simulink model "power_supply_test"  (R2025b)
settings: Solver=FixedStepAuto  StartTime=0.0  StopTime=2  RelTol=1e-3
model workspace (MAT data in the model file):
  Ap = 0.0314
  Ct = 2.4e-12
  Fforce = 90000
  GateChoice = "linear"
  Gmass = 9000
  K1 = 221320
  K2 = 0.00072
  Kc = 1.68e-09
  Kq = 1.63
  Ksvl = 0.0276
  Ksvr = 0.04
  U_PhaseRMS = 243
  Ve = 0.11304
  Xd = 0.003
  Xmax = 0.006
  Xmin = -0.004
  beta_e = 700000000
  delay_t = 1e-06
  dl = -0.014
  dr = 0.014
  k = 0.15
  lambda = 2
  rd = 0.0004
undefined symbols (not defined in the file or in its folder): R_rms, Rn_SNR, Ts_meas
libraries: ee_lib x13, nesl_utility x4, fl_lib x3, eeRmsMeasurement x3, simulink x1
settings Model: DataDictionary=ctrlSys.sldd  Creator=LYG  LastModifiedBy=LYG
settings SolverCC: ZeroCrossControl=DisableAll

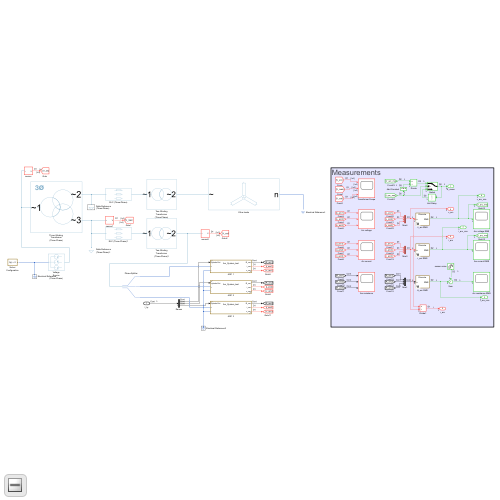
[thumbnail: Simulink's stored preview of the top-level diagram]
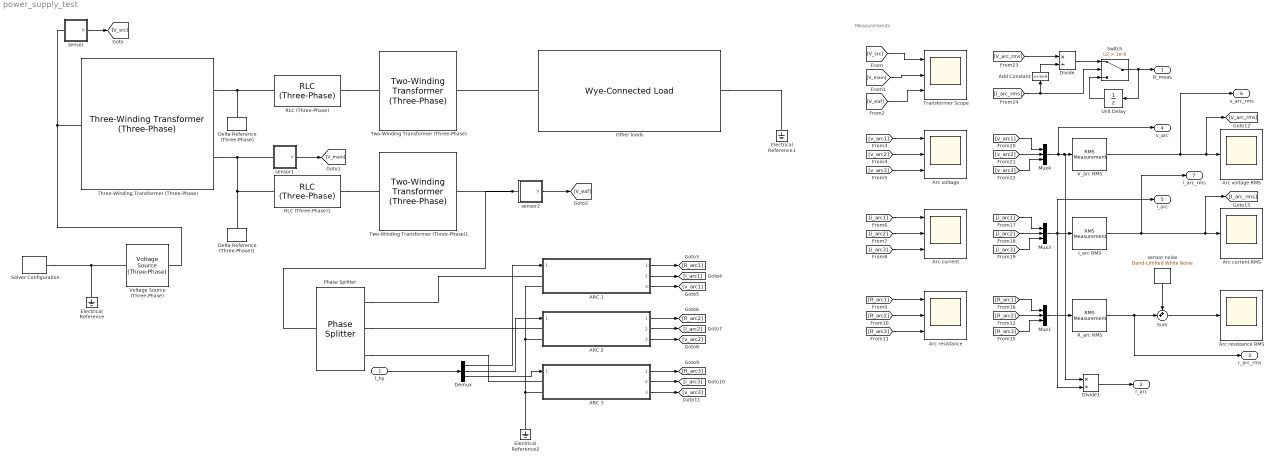
== system power_supply_test ==
  note: Measurements
  l_hy : Inport
  ARC 1 : Subsystem  ReferencedSubsystem=Arc_System_test
  ARC 2 : Subsystem  ReferencedSubsystem=Arc_System_test
  ARC 3 : Subsystem  ReferencedSubsystem=Arc_System_test
  Add Constant : Bias  Bias=1e-6  SaturateOnIntegerOverflow=off
  Arc current : Scope  NumInputPorts=3
      settings: ActiveDisplayYMinimum=-41973.164268779663  ActiveDisplayYMaximum=41974.004776580055  DataLoggingVariableName=ScopeData2
  Arc current RMS : Scope
      settings: ActiveDisplayYMinimum=-3055.4847803654839  ActiveDisplayYMaximum=27499.363023289359  DataLoggingVariableName=ScopeData7
  Arc resistance : Scope  NumInputPorts=3
      settings: ActiveDisplayYMinimum=-0.1125194623785952  ActiveDisplayYMaximum=1.0569916577736953  DataLoggingVariableName=ScopeData3
  Arc resistance RMS : Scope
      settings: ActiveDisplayYMinimum=0.04995143409404143  ActiveDisplayYMaximum=0.074820253608208473  DataLoggingVariableName=ScopeData4
  Arc voltage : Scope  NumInputPorts=3
      settings: ActiveDisplayYMinimum=351.3925306602107  ActiveDisplayYMaximum=415.43919686304929
  Arc voltage RMS : Scope
      settings: ActiveDisplayYMinimum=-47.465203373542423  ActiveDisplayYMaximum=427.18683036188185  DataLoggingVariableName=ScopeData8
  Delta Reference (Three-Phase) : ee_lib/Connectors & References/Delta Reference (Three-Phase)
      settings: InternalSimscapePortConfiguration="{\"Bottom\":[],\"Left\":[{\"id\":\"N\",\"label\":\"~\",\"type\":\"foundation.electrical.three_phase\"}],\"Right\":[],\"Top\":[]}"
  Delta Reference (Three-Phase)1 : ee_lib/Connectors & References/Delta Reference (Three-Phase)
      settings: InternalSimscapePortConfiguration="{\"Bottom\":[],\"Left\":[{\"id\":\"N\",\"label\":\"~\",\"type\":\"foundation.electrical.three_phase\"}],\"Right\":[],\"Top\":[]}"
  Demux : Demux  Outputs=3
  Divide : Product  Inputs=*/  OutMin=0
  Divide1 : Product  Inputs=*/
  Electrical Reference : fl_lib/Electrical/Electrical Elements/Electrical Reference
  Electrical Reference1 : fl_lib/Electrical/Electrical Elements/Electrical Reference
  Electrical Reference2 : fl_lib/Electrical/Electrical Elements/Electrical Reference
  I_arc RMS : eeRmsMeasurement/RMS Measurement  LabelModeActiveChoice=Total  F=f  SpecifyHarmonics=off  K=[0 1 2]  Ts=Ts_meas
      settings: LibrarySourceBlock=|
      | ee_sl_lib/Measurements/RMS
      | Measurement
  Mux1 : Mux  Inputs=3
  Mux3 : Mux  Inputs=3
  Mux4 : Mux  Inputs=3
  Other loads : ee_lib/Passive/RLC Assemblies/Wye-Connected Load  port_option=ee.enum.threePhasePort.composite  parameterization=ee.enum.rlc.parameterization.ratedpower  component_structure=ee.enum.rlc.structure.R  component_structure_PQ=ee.enum.rlc.structure.SeriesRLC  R=1 Ohm  L=1e-3 H  C=1e-6 F  VRated=6000 V  FRated=f Hz  P=10000 W  Qpos=100 A*V  Qneg=-1e2 A*V  R_parasitic=0 Ohm  G_parasitic=0 1/Ohm  R_parasitic_PQ=0 Ohm  G_parasitic_PQ=0 1/Ohm  Vmag0=24e3 V  Vang0=0 deg  Freq0=60 Hz  IL_specify=off  IL_priority=High  IL=[0, 0, 0] A  IL_nominal_specify=off  IL_nominal_value=1  IL_nominal_unit=A  VC_specify=off  VC_priority=High  VC=[0, 0, 0] V  VC_nominal_specify=off  VC_nominal_value=1  VC_nominal_unit=V
  Phase Splitter : ee_lib/Connectors & References/Phase Splitter
  RLC (Three-Phase) : ee_lib/Passive/RLC Assemblies/RLC (Three-Phase)  port_option=ee.enum.threePhasePort.composite  component_structure=ee.enum.rlc.structure.R  R=0.256 Ohm  L=8e-3 H  C=1e-6 F  R_parasitic=0 Ohm  G_parasitic=0 1/Ohm  IL_specify=off  IL_priority=High  IL=[0, 0, 0] A  IL_nominal_specify=off  IL_nominal_value=1  IL_nominal_unit=A  VC_specify=off  VC_priority=High  VC=[0, 0, 0] V  VC_nominal_specify=off  VC_nominal_value=1  VC_nominal_unit=V
      settings: InternalSimscapePortConfiguration="{\"Bottom\":[],\"Left\":[{\"id\":\"N1\",\"label\":\"~1\",\"type\":\"foundation.electrical.three_phase\"}],\"Right\":[{\"id\":\"N2\",\"label\":\"~2\",\"type\":\"foundation.electrical.three_phase\"}],\"Top\":[]}"
  RLC (Three-Phase)1 : ee_lib/Passive/RLC Assemblies/RLC (Three-Phase)  port_option=ee.enum.threePhasePort.composite  component_structure=ee.enum.rlc.structure.R  R=0.256 Ohm  L=8e-3 H  C=1e-6 F  R_parasitic=0 Ohm  G_parasitic=0 1/Ohm  IL_specify=off  IL_priority=High  IL=[0, 0, 0] A  IL_nominal_specify=off  IL_nominal_value=1  IL_nominal_unit=A  VC_specify=off  VC_priority=High  VC=[0, 0, 0] V  VC_nominal_specify=off  VC_nominal_value=1  VC_nominal_unit=V
      settings: InternalSimscapePortConfiguration="{\"Bottom\":[],\"Left\":[{\"id\":\"N1\",\"label\":\"~1\",\"type\":\"foundation.electrical.three_phase\"}],\"Right\":[{\"id\":\"N2\",\"label\":\"~2\",\"type\":\"foundation.electrical.three_phase\"}],\"Top\":[]}"
  R_arc RMS : eeRmsMeasurement/RMS Measurement  LabelModeActiveChoice=Total  F=f  SpecifyHarmonics=off  K=[0 1 2]  Ts=Ts_meas
      settings: LibrarySourceBlock=|
      | ee_sl_lib/Measurements/RMS
      | Measurement
  Solver Configuration : nesl_utility/Solver Configuration  PhysicalDomain=network_engine_domain  SubClassName=solver  LeftPortType=input  RightPortType=generic  Tones=[]  Harmonics=[]  SimulateNoise=off  Profile=off  UseLocalSampling=off  EnableSwitchedLinearOptims=on  FrequencyDomain=off  UseCCode=off  RelTol=0.001  AbsTol=0.001  MinStep=1e-09  ToWorkspace=off  RevertToSquareIcSolve=off  NumHomotopyIterations=100  PhasorMode=off  PhasorModeNumHarmonics=1  ConsistencySolver=NEWTON_XTOL_AFTER_FTOL  IndexReductionMethod=DerivativeReplacement  DoDC=off  ResidualTolerance=1e-09  ConsistencyTolSource=GLOBAL  ConsistencyAbsTol=0.001  ConsistencyRelTol=0.001  ConsistencyTolFactor=0.001  UseLocalSolver=on  LocalSolverChoice=NE_BACKWARD_EULER_ADVANCER  ResolveIndetEquations=on  FunctionEvalNumThread=1  LocalSolverSampleTime=Ts_local  DoFixedCost=off  MaxNonlinIter=5  MaxModeIter=2  ComputeImpulses=off  ImpulseIterations=2  LinearAlgebra=auto  LinearAlgebraNumThread=0  EquationFormulation=NE_TIME_EF  DelaysMemoryBudget=1024  AutomaticFiltering=on  FilteringTimeConstant=0.001  PartitionStorageMethod=AS_NEEDED  PartitionMemoryBudget=1024  PartitionMethod=ROBUST  MultibodyUseLocalSolver=off  MultibodyLocalSolverChoice=ODE1  MultibodyLocalSolverSampleTime=0.001
  Sum : Sum  Inputs=++|
  Switch : Switch  Criteria=u2 > Threshold  Threshold=1e-6  SaturateOnIntegerOverflow=off  InputSameDT=off
  Three-Winding Transformer (Three-Phase) : ee_lib/Passive/Transformers/Three-Winding Transformer (Three-Phase)  SRated=100e6 A*V  FRated=f Hz  Winding1Connection=ee.enum.windingconnection.delta1  VRated1=110e3 V  Winding2Connection=ee.enum.windingconnection.delta1  VRated2=3.5e3 V  Winding3Connection=ee.enum.windingconnection.delta1  VRated3=3.5e3 V  CoreType=ee.enum.coretype.threelimb  pu_Rw1=0.01  pu_Rw2=0.01  pu_Rw3=0.01  leakage_reactance_option=ee.enum.transformer_leakage.exclude  pu_Xl1=0.05  pu_Xl2=0.05  pu_Xl3=0.05  magnetizing_resistance_option=ee.enum.transformer_magnetizingResistance.exclude  pu_Rm=500  magnetizing_reactance_option=ee.enum.transformer_magnetizingReactance.exclude  saturation_option=ee.enum.transformer_saturation.exclude  pu_Xm=500  current_data=[0, .002, 1, 2]  magnetic_flux_data=[0, 1.2, 1.5, 1.51]  pu_X0=0.5  i1_specify=off  i1_priority=None  i1=[0, 0, 0] A  i1_nominal_specify=off  i1_nominal_value=1  i1_nominal_unit=A  i2_specify=off  i2_priority=None  i2=[0, 0, 0] A  i2_nominal_specify=off  i2_nominal_value=1  i2_nominal_unit=A  i3_specify=off  i3_priority=None  i3=[0, 0, 0] A  i3_nominal_specify=off  i3_nominal_value=1  i3_nominal_unit=A  phi_specify=off  phi_priority=None  phi=[0, 0, 0]  phi_nominal_specify=off  phi_nominal_value=1  phi_nominal_unit=1  power_dissipated_specify=off  power_dissipated_priority=None  power_dissipated=0 W  power_dissipated_nominal_specify=off  power_dissipated_nominal_value=1  power_dissipated_nominal_unit=W
      settings: InternalSimscapePortConfiguration="{\"Bottom\":[],\"Left\":[{\"id\":\"N1\",\"label\":\"~1\",\"type\":\"foundation.electrical.three_phase\"}],\"Right\":[{\"id\":\"N2\",\"label\":\"~2\",\"type\":\"foundation.electrical.three_phase\"},{\"id\":\"N3\",\"label\":\"~3\",\"type\":\"foundation.electrical.three_phase\"}],\"Top\":[]}"
  Transformer Scope : Scope  NumInputPorts=3
      settings: ActiveDisplayYMinimum=-194454.28422245517  ActiveDisplayYMaximum=194453.63939169198
  Two-Winding Transformer (Three-Phase) : ee_lib/Passive/Transformers/Two-Winding Transformer (Three-Phase)  SRated=100e6 A*V  FRated=f Hz  Winding1Connection=ee.enum.windingconnection.delta1  VRated1=735000 V  Winding2Connection=ee.enum.windingconnection.Y  VRated2=8820 V  CoreType=ee.enum.coretype.threelimb  pu_Rw1=0.01  pu_Rw2=0.01  leakage_reactance_option=ee.enum.transformer_leakage.exclude  pu_Xl1=0.05  pu_Xl2=0.05  magnetizing_resistance_option=ee.enum.transformer_magnetizingResistance.exclude  pu_Rm=500  magnetizing_reactance_option=ee.enum.transformer_magnetizingReactance.exclude  saturation_option=ee.enum.transformer_saturation.exclude  pu_Xm=500  current_data=[0, .002, 1, 2]  magnetic_flux_data=[0, 1.2, 1.5, 1.51]  pu_X0=0.5  i1_specify=off  i1_priority=None  i1=[0, 0, 0] A  i1_nominal_specify=off  i1_nominal_value=1  i1_nominal_unit=A  i2_specify=off  i2_priority=None  i2=[0, 0, 0] A  i2_nominal_specify=off  i2_nominal_value=1  i2_nominal_unit=A  phi_specify=off  phi_priority=None  phi=[0, 0, 0]  phi_nominal_specify=off  phi_nominal_value=1  phi_nominal_unit=1  power_dissipated_specify=off  power_dissipated_priority=None  power_dissipated=0 W  power_dissipated_nominal_specify=off  power_dissipated_nominal_value=1  power_dissipated_nominal_unit=W
      settings: InternalSimscapePortConfiguration="{\"Bottom\":[],\"Left\":[{\"id\":\"N1\",\"label\":\"~1\",\"type\":\"foundation.electrical.three_phase\"}],\"Right\":[{\"id\":\"N2\",\"label\":\"~2\",\"type\":\"foundation.electrical.three_phase\"}],\"Top\":[]}"
  Two-Winding Transformer (Three-Phase)1 : ee_lib/Passive/Transformers/Two-Winding Transformer (Three-Phase)  SRated=100e6 A*V  FRated=f Hz  Winding1Connection=ee.enum.windingconnection.delta1  VRated1=3.5e3 V  Winding2Connection=ee.enum.windingconnection.delta1  VRated2=580 V  CoreType=ee.enum.coretype.threelimb  pu_Rw1=0.01  pu_Rw2=0.01  leakage_reactance_option=ee.enum.transformer_leakage.exclude  pu_Xl1=0.05  pu_Xl2=0.05  magnetizing_resistance_option=ee.enum.transformer_magnetizingResistance.exclude  pu_Rm=500  magnetizing_reactance_option=ee.enum.transformer_magnetizingReactance.exclude  saturation_option=ee.enum.transformer_saturation.exclude  pu_Xm=500  current_data=[0, .002, 1, 2]  magnetic_flux_data=[0, 1.2, 1.5, 1.51]  pu_X0=0.5  i1_specify=off  i1_priority=None  i1=[0, 0, 0] A  i1_nominal_specify=off  i1_nominal_value=1  i1_nominal_unit=A  i2_specify=off  i2_priority=None  i2=[0, 0, 0] A  i2_nominal_specify=off  i2_nominal_value=1  i2_nominal_unit=A  phi_specify=off  phi_priority=None  phi=[0, 0, 0]  phi_nominal_specify=off  phi_nominal_value=1  phi_nominal_unit=1  power_dissipated_specify=off  power_dissipated_priority=None  power_dissipated=0 W  power_dissipated_nominal_specify=off  power_dissipated_nominal_value=1  power_dissipated_nominal_unit=W
      settings: InternalSimscapePortConfiguration="{\"Bottom\":[],\"Left\":[{\"id\":\"N1\",\"label\":\"~1\",\"type\":\"foundation.electrical.three_phase\"}],\"Right\":[{\"id\":\"N2\",\"label\":\"~2\",\"type\":\"foundation.electrical.three_phase\"}],\"Top\":[]}"
  Unit Delay : UnitDelay  SampleTime=-1  HasFrameUpgradeWarning=on
  V_arc RMS : eeRmsMeasurement/RMS Measurement  LabelModeActiveChoice=Total  F=f  SpecifyHarmonics=off  K=[0 1 2]  Ts=Ts_meas
      settings: LibrarySourceBlock=|
      | ee_sl_lib/Measurements/RMS
      | Measurement
  Voltage Source (Three-Phase) : ee_lib/Sources/Voltage Source (Three-Phase)  vline_rms=110e3 V  shift=0 deg  freq=f Hz  impedance_option=0  SShortCircuit=1e6 A*V  XR=15  R=0.01 Ohm  L=3.97e-4 H  harmonic_option=0  harmonic_orders=[5, 7, 11, 13]  harmonic_ratios=[.1, .1, .1, .1]  G_parasitic=0 1/Ohm  I_specify=off  I_priority=None  I=[0, 0, 0] A  I_nominal_specify=off  I_nominal_value=1  I_nominal_unit=A
  sensor : Subsystem
  sensor noise : simulink/Sources/Band-Limited White Noise  Cov=Ts_meas * (R_rms / (10^(Rn_SNR / 20)))^2  Ts=Ts_meas  seed=Rn_seed
  sensor1 : Subsystem
  sensor2 : Subsystem
  R_meas : Outport
  r_arc : Outport  Port=2
  r_arc_rms : Outport  Port=3
  v_arc : Outport  Port=4
  i_arc : Outport  Port=5
  v_arc_rms : Outport  Port=6
  i_arc_rms : Outport  Port=7
  wires:
  [V_src] -> Transformer Scope/1
  sensor/1(V) -> [V_src]
  sensor1/1(V) -> [V_main]
  [V_main] -> Transformer Scope/2
  sensor2/1(V) -> [V_eaf]
  [V_eaf] -> Transformer Scope/3
  ARC 1/1 -> [R_arc1]
  ARC 1/2 -> [i_arc1]
  ARC 1/3 -> [v_arc1]
  ARC 2/3 -> [v_arc2]
  ARC 2/2 -> [i_arc2]
  ARC 2/1 -> [R_arc2]
  ARC 3/1 -> [R_arc3]
  ARC 3/2 -> [i_arc3]
  ARC 3/3 -> [v_arc3]
  [v_arc1] -> Arc voltage/1
  [v_arc2] -> Arc voltage/2
  [v_arc3] -> Arc voltage/3
  [i_arc1] -> Arc current/1
  [i_arc2] -> Arc current/2
  [i_arc3] -> Arc current/3
  Demux/1 -> ARC 1/1
  Demux/2 -> ARC 2/1
  Demux/3 -> ARC 3/1
  Mux3/1 -> Divide1/2, i_arc/1, I_arc RMS/1
  Mux4/1 -> Divide1/1, V_arc RMS/1, v_arc/1
  [i_arc1] -> Mux3/1
  [i_arc2] -> Mux3/2
  [i_arc3] -> Mux3/3
  I_arc RMS/1 -> i_arc_rms/1, [I_arc_rms], Arc current RMS/1
  [v_arc1] -> Mux4/1
  [v_arc2] -> Mux4/2
  [v_arc3] -> Mux4/3
  V_arc RMS/1 -> v_arc_rms/1, [V_arc_rms], Arc voltage RMS/1
  Switch/1 -> R_meas/1, Unit Delay/1
  Add Constant/1 -> Divide/2
  [V_arc_rms] -> Divide/1
  [I_arc_rms] -> Switch/2, Add Constant/1
  Divide/1 -> Switch/1
  Unit Delay/1 -> Switch/3
  [R_arc1] -> Mux1/1
  [R_arc3] -> Arc resistance/3
  Mux1/1 -> R_arc RMS/1
  [R_arc2] -> Mux1/2
  [R_arc3] -> Mux1/3
  [R_arc1] -> Arc resistance/1
  [R_arc2] -> Arc resistance/2
  Sum/1 -> Arc resistance RMS/1
  sensor noise/1 -> Sum/1
  R_arc RMS/1 -> r_arc_rms/1, Sum/2
  l_hy/1 -> Demux/1
  Divide1/1 -> r_arc/1
  connections:
  Three-Winding Transformer (Three-Phase)/LConn1 -- sensor/LConn1 -- Voltage Source (Three-Phase)/RConn1
  Other loads/LConn1 -- Two-Winding Transformer (Three-Phase)/RConn1
  RLC (Three-Phase)/RConn1 -- Two-Winding Transformer (Three-Phase)/LConn1
  RLC (Three-Phase)1/RConn1 -- Two-Winding Transformer (Three-Phase)1/LConn1
  Three-Winding Transformer (Three-Phase)/RConn2 -- sensor1/LConn1 -- RLC (Three-Phase)1/LConn1 -- Delta Reference (Three-Phase)1/LConn1
  Three-Winding Transformer (Three-Phase)/RConn1 -- RLC (Three-Phase)/LConn1 -- Delta Reference (Three-Phase)/LConn1
  sensor2/LConn1 -- Two-Winding Transformer (Three-Phase)1/RConn1 -- Phase Splitter/LConn1
  Phase Splitter/RConn1 -- ARC 1/LConn1
  Phase Splitter/RConn2 -- ARC 2/LConn1
  Phase Splitter/RConn3 -- ARC 3/LConn1
  Other loads/RConn1 -- Electrical Reference1/LConn1
  ARC 1/LConn2 -- ARC 2/LConn2 -- ARC 3/LConn2 -- Electrical Reference2/LConn1
  Solver Configuration/RConn1 -- Electrical Reference/LConn1 -- Voltage Source (Three-Phase)/LConn1

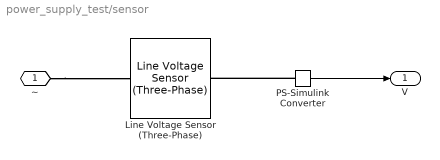
== system power_supply_test/sensor ==
  Line Voltage Sensor (Three-Phase) : ee_lib/Sensors & Transducers/Line Voltage Sensor (Three-Phase)
  PS-Simulink Converter : nesl_utility/PS-Simulink Converter  PhysicalDomain=network_engine_domain  SubClassName=ps_output  LeftPortType=input  RightPortType=output  PseudoPeriodic=off  Frequencies=[]  VectorFormat=inherit  Unit=inherit  AffineConversion=off
  ~ : PMIOPort  Side=Left
  V : Outport
  wires:
  PS-Simulink Converter/1 -> V/1
  connections:
  ~/RConn1 -- Line Voltage Sensor (Three-Phase)/LConn1
  PS-Simulink Converter/LConn1 -- Line Voltage Sensor (Three-Phase)/RConn1

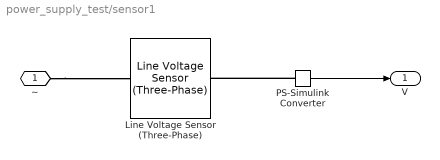
== system power_supply_test/sensor1 ==
  Line Voltage Sensor (Three-Phase) : ee_lib/Sensors & Transducers/Line Voltage Sensor (Three-Phase)
  PS-Simulink Converter : nesl_utility/PS-Simulink Converter  PhysicalDomain=network_engine_domain  SubClassName=ps_output  LeftPortType=input  RightPortType=output  PseudoPeriodic=off  Frequencies=[]  VectorFormat=inherit  Unit=inherit  AffineConversion=off
  ~ : PMIOPort  Side=Left
  V : Outport
  wires:
  PS-Simulink Converter/1 -> V/1
  connections:
  ~/RConn1 -- Line Voltage Sensor (Three-Phase)/LConn1
  PS-Simulink Converter/LConn1 -- Line Voltage Sensor (Three-Phase)/RConn1

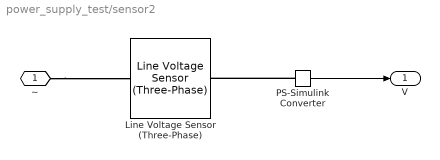
== system power_supply_test/sensor2 ==
  Line Voltage Sensor (Three-Phase) : ee_lib/Sensors & Transducers/Line Voltage Sensor (Three-Phase)
  PS-Simulink Converter : nesl_utility/PS-Simulink Converter  PhysicalDomain=network_engine_domain  SubClassName=ps_output  LeftPortType=input  RightPortType=output  PseudoPeriodic=off  Frequencies=[]  VectorFormat=inherit  Unit=inherit  AffineConversion=off
  ~ : PMIOPort  Side=Left
  V : Outport
  wires:
  PS-Simulink Converter/1 -> V/1
  connections:
  PS-Simulink Converter/LConn1 -- Line Voltage Sensor (Three-Phase)/RConn1
  ~/RConn1 -- Line Voltage Sensor (Three-Phase)/LConn1
